simulink model "Bebop7_like6_but_spline_only_from_SP"  (R2018a)
settings: Solver=VariableStepAuto  StartTime=0.0  StopTime=20  FixedStep=.04  MaxStep=1.00  MinStep=0.005  RelTol=10  AbsTol=10
values from neighbouring files (symbols this model uses):
  flightplan = [dist,0,height,deg2rad(090) ... (first row only)    [compare_cubic_spline_1.m]    (also in initialize_race_realtime.m; initialize_race_realtime_backup_cubic.m; plot_sim.m = [ 4.348, -0.278, height, deg2rad(  0); test_b_spline.m)
  FOV = 1.05    [initialize_race_realtime.m]    (also in initialize_race_realtime_backup_cubic.m)
  g = 9.81    [initialize_race_no_realtime.m]    (also in initialize_race_realtime.m; initialize_race_realtime_backup_cubic.m; moving_average_rls_own.m = P(i-1)*meas*(lambda+meas*P(i-1)*meas)^-1)
  gate_size = 1.4    [initialize_race_realtime.m]    (also in initialize_race_realtime_backup_cubic.m)
  gates = sim_gates(:,:,1)    [eval_sim.m]    (also in initialize_race_realtime.m = [dist,0,height,deg2rad(110); initialize_race_realtime_backup_cubic.m = [dist,0,height,deg2rad(110); plot_sim.m)
  I = [1 0 0 ... (first row only)    [Bebop_sim_init.m]    (also in initialize_race_no_realtime.m; initialize_race_realtime.m; initialize_race_realtime_backup_cubic.m; moving_averge_rls_download.m = ones(1,N))
  init_std_dev = [1.0*ones(1,3),deg2rad(30)]    [initialize_race_realtime.m]    (also in initialize_race_realtime_backup_cubic.m)
  m = 0.68    [calc_plot_spline.m]    (also in calc_spline.m; compare_cubic_spline_1.m = vpasolve(e,r); compare_cubic_spline_2.m = r/3*(-sin(dp)+sqrt(sin(dp)^2-6*cos(dp)+6)); initialize_race_no_realtime.m = 2)
  max_rot_Z = (90)*pi/180    (= 1.57079632679)    [Bebop_sim_init.m]    (also in initialize_race_no_realtime.m = 1.0471975512; initialize_race_realtime.m; initialize_race_realtime_backup_cubic.m; run_batch1.m = list_agility(idx_agility)*max_rot_Z)
  max_theta_X = (40)*pi/180    (= 0.698131700798)    [Bebop_sim_init.m]    (also in initialize_race_no_realtime.m = 0.13962634016; initialize_race_realtime.m = 1.308996939; initialize_race_realtime_backup_cubic.m = 1.308996939; run_batch1.m = list_agility(idx_agility)*max_theta_X)
  max_theta_Y = (40)*pi/180    (= 0.698131700798)    [Bebop_sim_init.m]    (also in initialize_race_no_realtime.m = 0.13962634016; initialize_race_realtime.m = 1.308996939; initialize_race_realtime_backup_cubic.m = 1.308996939; run_batch1.m = list_agility(idx_agility)*max_theta_Y)
  max_v_Z = .5    (= 0.5)    [Bebop_sim_init.m]    (also in initialize_race_no_realtime.m = 1; initialize_race_realtime.m = 3; initialize_race_realtime_backup_cubic.m = 3; run_batch1.m = list_agility(idx_agility)*max_v_Z)
  max_vel = 1.5    [initialize_race_realtime.m]    (also in initialize_race_realtime_backup_cubic.m; run_batch1.m = list_speed(idx_speed); run_batch2.m = list_speed(idx_speed); run_batch3.m = list_speed(idx_speed))
  spline_init = [P0;P1;P2;P3]    [initialize_race_realtime.m]
  std_dev_factor = 1.0    (= 1)    [initialize_race_realtime.m]
  std_dev_switch = std_dev_factor/5    (= 0.2)    [initialize_race_realtime.m]
undefined symbols (not defined in the file or in its folder): fspecial, gray, Rec, SDTV
libraries: simulink x11, sharedtransform x11, visionanalysis x7, visiontextngfix x5, visiontransforms x3, aerolibactuator x2, aerolibutil x2, visionstatistics x2, visionconversions x2, shared6dof x1, vrlib x1, visionsinks x1
(part 1 of 3)
settings Model: EnablePacing=on  Creator=vinni  LastModifiedBy=lenny
settings SolverCC: MaxConsecutiveMinStep=99999  ShapePreserveControl=EnableAll  ZeroCrossAlgorithm=Adaptive
settings DebuggingCC: WriteAfterWriteMsg=EnableAllAsError  AlgebraicLoopMsg=error  IntegerOverflowMsg=error  ParameterUnderflowMsg=error  UniqueDataStoreMsg=error  NonBusSignalsTreatedAsBus=error  IntegerSaturationMsg=error
settings HardwareCC: ProdBitPerLong=64  ProdHWDeviceType=Intel->x86-64 (Linux 64)

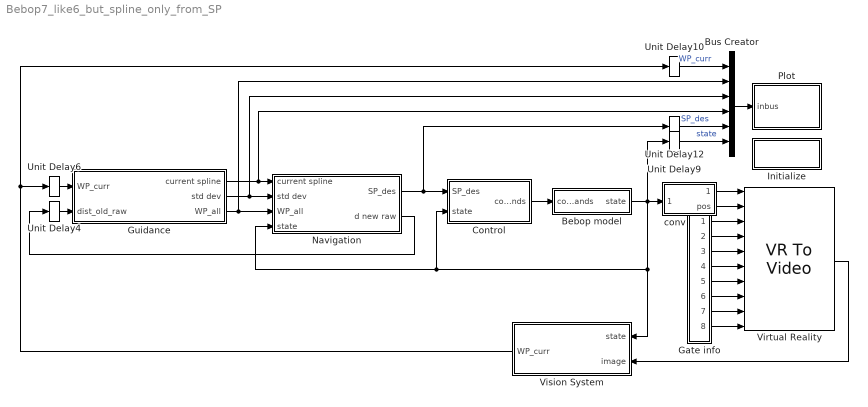
== system Bebop7_like6_but_spline_only_from_SP ==
  Bebop model : Subsystem
  Bus Creator : BusCreator  Inputs=6  OutDataTypeStr=Bus: PlotBus  NonVirtualBus=on
  Control : Subsystem
  Gate info : Subsystem
  Guidance : Subsystem
  Initialize : Subsystem  TreatAsAtomicUnit=on
  Navigation : Subsystem
  Plot : MATLAB Function  TreatAsAtomicUnit=on
  Unit Delay{4,6,9..10,12} (5 alike) : UnitDelay  SampleTime=-1
  Virtual Reality : vrlib/VR To Video  InstantiateOnLoad=on  SampleTime=0.075  ViewEnable=on  RemoteChange=off  RemoteView=off  FieldsWritten=drone.orientation.4.1.1.double#drone.position.3.1.1.double#G1.rotation.4.1.1.double#G1.translation.3.1.1.double#G2.rotation.4.1.1.double#G2.translation.3.1.1.double#G3.rotation.4.1.1.double#G3.translation.3.1.1.double#G4.rotation.4.1.1.double#G4.translation.3.1.1.double  WorldFileName=race_course.wrl  AutoView=off  VideoDimensions=1.5*[200 320]  AllowVariableSize=off  FigureProperties="{'Position', 'Name', 'Viewpoint', 'CameraBound', 'CameraDirection', 'CameraPosition', 'CameraUpVector', 'ZoomFactor', 'Antialiasing', 'Headlight', 'Lighting', 'NavPanel', 'Sound', 'StatusBar', 'Stereo3D', 'Stereo3DCameraOffset', 'Stereo3DHIT', 'ToolBar', 'Textures', 'Transparency', 'Triad', 'Wireframe', 'NavZones', 'NavMode', 'NavSpeed', 'CaptureFileFormat', 'CaptureFileName', 'Record2DCompressMethod', 'Record2DCompressQuality', 'Record2D', 'Record2DFileName', 'Record2DFPS'; [3.0000000000000000e+01   6.0000000000000000e+01   4.8000000000000000e+02   3.0000000000000000e+02], '', '_untitled_1', 'on', [0.0000000000000000e+00   0.0000000000000000e+00  -1.0000000000000000e+00], [0.0000000000000000e+00   0.0000000000000000e+00   0.0000000000000000e+00], [0.0000000000000000e+00   1.0000000000000000e+00   0.0000000000000000e+00], [1.0000000000000000e+00], 'on', 'on', 'on', 'none', 'on', 'off', 'off', [1.0000000149011612e-01], [0.0000000000000000e+00], 'off', 'on', 'on', 'none', 'off', 'off', 'fly', 'normal', 'tif', '%f_anim_%n.tif', 'auto', [7.5000000000000000e+01], 'off', '***video***', 'auto'}"
      settings: SourceProductName=Simulink 3D Animation  SourceProductBaseCode=VR
  Vision System : Subsystem
  conv : Subsystem
  wires:
  Vision System/1(WP_curr) -> Unit Delay10/1, Unit Delay6/1
  Virtual Reality/1 -> Vision System/2(image)
  Control/1(commands) -> Bebop model/1(commands)
  Unit Delay6/1 -> Guidance/1(WP_curr)
  Unit Delay4/1 -> Guidance/2(dist_old_raw)
  conv/1(axang) -> Virtual Reality/1
  Gate info/2(P1) -> Virtual Reality/4
  Gate info/4(P2) -> Virtual Reality/6
  Gate info/6(P3) -> Virtual Reality/8
  Gate info/8(P4) -> Virtual Reality/10
  Gate info/1(O1) -> Virtual Reality/3
  Gate info/3(O2) -> Virtual Reality/5
  Gate info/5(O3) -> Virtual Reality/7
  Gate info/7(O4) -> Virtual Reality/9
  Navigation/1(SP_des) -> Unit Delay12/1, Control/1(SP_des)
  Navigation/2(d new raw) -> Unit Delay4/1
  Bebop model/1(state) -> Vision System/1(state), Control/2(state), Navigation/4(state), Unit Delay9/1, conv/1(state)
  Bus Creator/1 -> Plot/1(inbus)
  Guidance/3(WP_all) -> Bus Creator/2, Navigation/3(WP_all)
  Guidance/2(std dev) -> Bus Creator/3, Navigation/2(std dev)
  Unit Delay9/1 -> Bus Creator/6  "state"
  Unit Delay10/1 -> Bus Creator/1  "WP_curr"
  Unit Delay12/1 -> Bus Creator/5  "SP_des"
  Guidance/1(current spline) -> Navigation/1(current spline), Bus Creator/4
  conv/2(pos) -> Virtual Reality/2

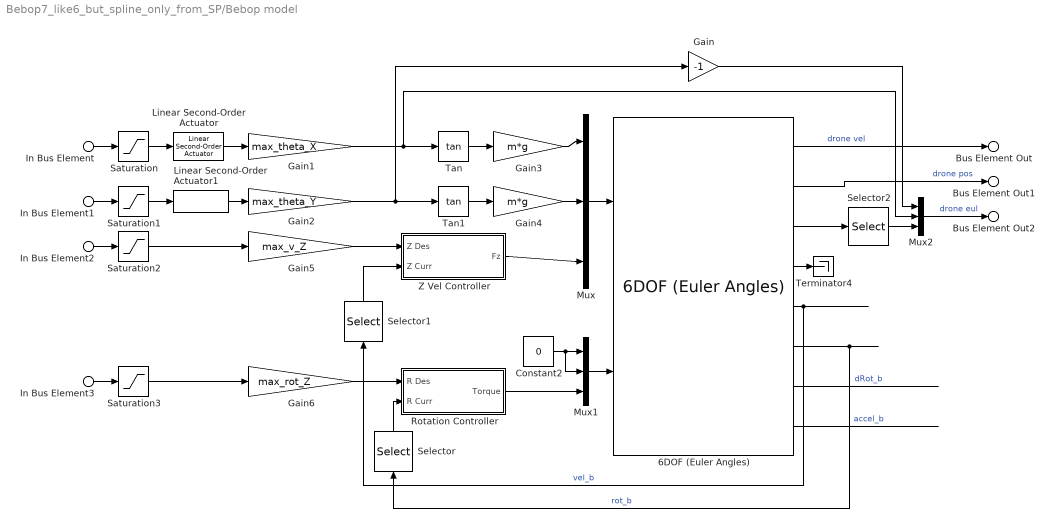
== system Bebop7_like6_but_spline_only_from_SP/Bebop model ==
  In Bus Element : Inport  PortName=commands  Element=pitch
  In Bus Element1 : Inport  PortName=commands  Element=roll
  In Bus Element2 : Inport  PortName=commands  Element=throttle
  In Bus Element3 : Inport  PortName=commands  Element=yaw
  6DOF (Euler Angles) : shared6dof/6DOF (Euler Angles)  units=Metric (MKS)  mtype=Fixed  rep=Euler Angles  xme_0=Initial_pos  Vm_0=Initial_vel_b  eul_0=Initial_ori  pm_0=[0 0 0]  mass_0=m  mass_e=0.5  mass_f=2.0  inertia=I  inertia_e=eye(3)  inertia_f=2*eye(3)  k_quat=1.0  vre_flag=on  abi_flag=off  aMode=0
      settings: SourceProductBaseCode=AE
  Constant2 : Constant  Value=0
  Gain : Gain  Gain=-1
  Gain1 : Gain  Gain=max_theta_X
  Gain2 : Gain  Gain=max_theta_Y
  Gain3 : Gain  Gain=m*g
  Gain4 : Gain  Gain=m*g
  Gain5 : Gain  Gain=max_v_Z
  Gain6 : Gain  Gain=max_rot_Z
  Linear Second-Order Actuator : aerolibactuator/Linear Second-Order Actuator  wn_fin=20  z_fin=1  fin_act_0=0  fin_act_vel=0
      settings: SourceProductName=Aerospace Blockset  SourceProductBaseCode=AE
  Linear Second-Order Actuator1 : aerolibactuator/Linear Second-Order Actuator  wn_fin=20  z_fin=1  fin_act_0=0  fin_act_vel=0
      settings: SourceProductName=Aerospace Blockset  SourceProductBaseCode=AE
  Mux : Mux  Inputs=3
  Mux1 : Mux  Inputs=3
  Mux2 : Mux  Inputs=3
  Rotation Controller : Subsystem
  Saturation{,1..3} (4 alike) : Saturate  UpperLimit=1  LowerLimit=-1
  Selector : Selector  InputPortWidth=3  IndexOptions=Index vector (dialog)  Indices=3  OutputSizes=1
  Selector1 : Selector  InputPortWidth=3  IndexOptions=Index vector (dialog)  Indices=3  OutputSizes=1
  Selector2 : Selector  InputPortWidth=3  IndexOptions=Index vector (dialog)  Indices=3  OutputSizes=1
  Tan : Trigonometry  Operator=tan
  Tan1 : Trigonometry  Operator=tan
  Terminator4 : Terminator
  Z Vel Controller : Subsystem
  Bus Element Out : Outport  PortName=state  Element=vel
  Bus Element Out1 : Outport  PortName=state  Element=pos
  Bus Element Out2 : Outport  PortName=state  Element=eul
  wires:
  6DOF (Euler Angles)/5 -> Selector1/1  "vel_b"
  Saturation/1 -> Linear Second-Order Actuator/1
  Tan1/1 -> Gain4/1
  In Bus Element3/1 -> Saturation3/1
  Linear Second-Order Actuator1/1 -> Gain2/1
  6DOF (Euler Angles)/8 -> ?  "accel_b"
  Z Vel Controller/1(Fz) -> Mux/3
  6DOF (Euler Angles)/1 -> Bus Element Out/1  "drone vel"
  Rotation Controller/1(Torque) -> Mux1/3
  Selector/1 -> Rotation Controller/2(R Curr)
  Selector1/1 -> Z Vel Controller/2(Z Curr)
  Gain3/1 -> Mux/1
  Saturation1/1 -> Linear Second-Order Actuator1/1
  6DOF (Euler Angles)/3 -> Selector2/1
  In Bus Element2/1 -> Saturation2/1
  Gain1/1 -> Mux2/2, Tan/1
  Mux/1 -> 6DOF (Euler Angles)/1
  Gain5/1 -> Z Vel Controller/1(Z Des)
  In Bus Element1/1 -> Saturation1/1
  Tan/1 -> Gain3/1
  Gain/1 -> Mux2/1
  6DOF (Euler Angles)/4 -> Terminator4/1
  Constant2/1 -> Mux1/2, Mux1/1
  Saturation2/1 -> Gain5/1
  Gain2/1 -> Tan1/1, Gain/1
  Saturation3/1 -> Gain6/1
  Linear Second-Order Actuator/1 -> Gain1/1
  Mux1/1 -> 6DOF (Euler Angles)/2
  Gain6/1 -> Rotation Controller/1(R Des)
  Gain4/1 -> Mux/2
  In Bus Element/1 -> Saturation/1
  6DOF (Euler Angles)/6 -> Selector/1  "rot_b"
  6DOF (Euler Angles)/7 -> ?  "dRot_b"
  Selector2/1 -> Mux2/3
  6DOF (Euler Angles)/2 -> Bus Element Out1/1  "drone pos"
  Mux2/1 -> Bus Element Out2/1  "drone eul"

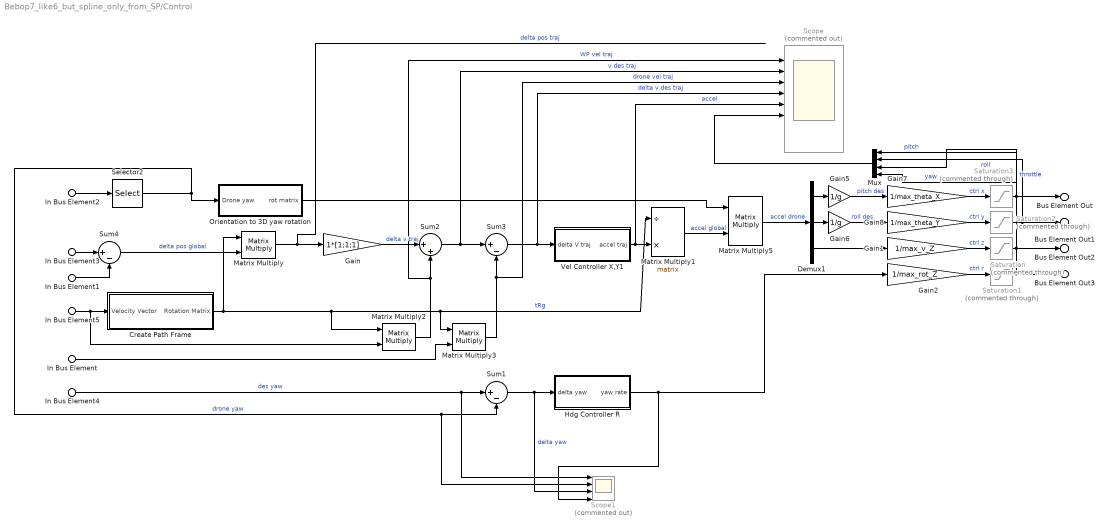
== system Bebop7_like6_but_spline_only_from_SP/Control ==
  In Bus Element5 : Inport  PortName=SP_des  Element=vel
  In Bus Element3 : Inport  PortName=SP_des  Element=pos
  In Bus Element4 : Inport  PortName=SP_des  Element=yaw
  In Bus Element : Inport  Port=2  PortName=state  Element=vel
  In Bus Element1 : Inport  Port=2  PortName=state  Element=pos
  In Bus Element2 : Inport  Port=2  PortName=state  Element=eul
  Create Path Frame : Subsystem
  Demux1 : Demux  Outputs=3
  Gain : Gain  Gain=1*[1;1;1]
  Gain1 : Gain  Gain=1/max_v_Z
  Gain2 : Gain  Gain=1/max_rot_Z
  Gain5 : Gain  Gain=1/g
  Gain6 : Gain  Gain=1/g
  Gain7 : Gain  Gain=1/max_theta_X
  Gain8 : Gain  Gain=1/max_theta_Y
  Hdg Controller R : Subsystem
  Matrix Multiply{,2..3,5} (4 alike) : Product  Inputs=**  Multiplication=Matrix(*)
  Matrix Multiply1 : Product  Inputs=/*  Multiplication=Matrix(*)
  Mux : Mux
  Orientation to 3D yaw rotation : Subsystem
  Saturation{,1..3} (4 alike) : Saturate  Commented=through  UpperLimit=1  LowerLimit=-1
  Scope : Scope  Commented=on  NumInputPorts=10
  Scope1 : Scope  Commented=on  NumInputPorts=4
  Selector2 : Selector  IndexMode=Zero-based  InputPortWidth=3  IndexOptions=Index vector (dialog)  Indices=2  OutputSizes=1
  Sum1 : Sum  Inputs=|+-
  Sum2 : Sum  Inputs=|++
  Sum3 : Sum  Inputs=|+-
  Sum4 : Sum  Inputs=|+-
  Vel Controller X,Y1 : Subsystem
  Bus Element Out : Outport  PortName=commands  Element=pitch
  Bus Element Out1 : Outport  PortName=commands  Element=roll
  Bus Element Out2 : Outport  PortName=commands  Element=throttle
  Bus Element Out3 : Outport  PortName=commands  Element=yaw
  wires:
  Saturation1/1 -> Bus Element Out3/1, Mux/4  "yaw"
  Saturation3/1 -> Bus Element Out/1, Mux/1  "pitch"
  Saturation2/1 -> Bus Element Out1/1, Mux/2  "roll"
  Saturation/1 -> Bus Element Out2/1, Mux/3  "throttle"
  In Bus Element4/1 -> Scope1/1, Sum1/1  "des yaw"
  In Bus Element3/1 -> Sum4/1
  In Bus Element5/1 -> Matrix Multiply2/2, Create Path Frame/1(Velocity Vector)
  Selector2/1 -> Scope1/2, Sum1/2, Orientation to 3D yaw rotation/1(Drone yaw)  "drone yaw"
  Gain7/1 -> Saturation3/1  "ctrl x"
  Demux1/3 -> Gain1/1
  Hdg Controller R/1(yaw rate) -> Scope1/4, Gain2/1
  Demux1/2 -> Gain6/1
  Mux/1 -> Scope/7
  Gain6/1 -> Gain8/1  "roll des"
  Sum3/1 -> Scope/5, Vel Controller X,Y1/1(delta V traj)  "delta v des traj"
  Matrix Multiply2/1 -> Scope/2, Sum2/2  "WP vel traj"
  Sum4/1 -> Matrix Multiply/2  "delta pos global"
  Matrix Multiply3/1 -> Scope/4, Sum3/2  "drone vel traj"
  Demux1/1 -> Gain5/1
  Gain1/1 -> Saturation/1  "ctrl z"
  Matrix Multiply/1 -> Gain/1  "delta pos traj"
  Gain5/1 -> Gain7/1  "pitch des"
  Vel Controller X,Y1/1(accel traj) -> Scope/6, Matrix Multiply1/2  "accel"
  Matrix Multiply5/1 -> Demux1/1  "accel drone"
  Orientation to 3D yaw rotation/1(rot matrix) -> Matrix Multiply5/1
  Gain8/1 -> Saturation2/1  "ctrl y"
  In Bus Element1/1 -> Sum4/2
  Create Path Frame/1(Rotation Matrix) -> Matrix Multiply/1, Matrix Multiply2/1, Matrix Multiply1/1, Matrix Multiply3/1  "tRg"
  Gain2/1 -> Saturation1/1  "ctrl r"
  In Bus Element/1 -> Matrix Multiply3/2
  Gain/1 -> Sum2/1  "delta v traj"
  Sum2/1 -> Scope/3, Sum3/1  "v des traj"
  Matrix Multiply1/1 -> Matrix Multiply5/2  "accel global"
  Sum1/1 -> Scope1/3, Hdg Controller R/1(delta yaw)  "delta yaw"
  In Bus Element2/1 -> Selector2/1

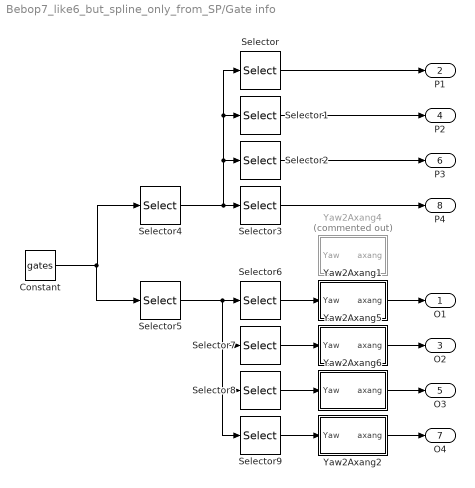
== system Bebop7_like6_but_spline_only_from_SP/Gate info ==
  Constant : Constant  Value=gates
  Selector : Selector  NumberOfDimensions=2  IndexMode=Zero-based  InputPortWidth=3  IndexOptions=Index vector (dialog),Select all  Indices=0,1  OutputSizes=1,1
  Selector1 : Selector  NumberOfDimensions=2  IndexMode=Zero-based  InputPortWidth=3  IndexOptions=Index vector (dialog),Select all  Indices=1,1  OutputSizes=1,1
  Selector2 : Selector  NumberOfDimensions=2  IndexMode=Zero-based  InputPortWidth=3  IndexOptions=Index vector (dialog),Select all  Indices=2,1  OutputSizes=1,1
  Selector3 : Selector  NumberOfDimensions=2  IndexMode=Zero-based  InputPortWidth=3  IndexOptions=Index vector (dialog),Select all  Indices=3,1  OutputSizes=1,1
  Selector4 : Selector  NumberOfDimensions=2  IndexMode=Zero-based  InputPortWidth=3  IndexOptions=Select all,Index vector (dialog)  Indices=4,[0 1 2]  OutputSizes=1,1
  Selector5 : Selector  NumberOfDimensions=2  IndexMode=Zero-based  InputPortWidth=3  IndexOptions=Select all,Index vector (dialog)  Indices=4,3  OutputSizes=1,1
  Selector6 : Selector  NumberOfDimensions=2  IndexMode=Zero-based  InputPortWidth=3  IndexOptions=Index vector (dialog),Select all  Indices=0,1  OutputSizes=1,1
  Selector7 : Selector  NumberOfDimensions=2  IndexMode=Zero-based  InputPortWidth=3  IndexOptions=Index vector (dialog),Select all  Indices=1,1  OutputSizes=1,1
  Selector8 : Selector  NumberOfDimensions=2  IndexMode=Zero-based  InputPortWidth=3  IndexOptions=Index vector (dialog),Select all  Indices=2,1  OutputSizes=1,1
  Selector9 : Selector  NumberOfDimensions=2  IndexMode=Zero-based  InputPortWidth=3  IndexOptions=Index vector (dialog),Select all  Indices=3,1  OutputSizes=1,1
  Yaw2Axang1 : Subsystem
  Yaw2Axang2 : Subsystem
  Yaw2Axang4 : Subsystem  Commented=on
  Yaw2Axang5 : Subsystem
  Yaw2Axang6 : Subsystem
  O1 : Outport
  P1 : Outport  Port=2
  O2 : Outport  Port=3
  P2 : Outport  Port=4
  O3 : Outport  Port=5
  P3 : Outport  Port=6
  O4 : Outport  Port=7
  P4 : Outport  Port=8
  wires:
  Selector/1 -> P1/1
  Selector3/1 -> P4/1
  Selector2/1 -> P3/1
  Selector4/1 -> Selector1/1, Selector/1, Selector2/1, Selector3/1
  Selector1/1 -> P2/1
  Constant/1 -> Selector5/1, Selector4/1
  Selector5/1 -> Selector9/1, Selector8/1, Selector7/1, Selector6/1
  Selector6/1 -> Yaw2Axang1/1(Yaw)
  Selector7/1 -> Yaw2Axang5/1(Yaw)
  Selector8/1 -> Yaw2Axang6/1(Yaw)
  Selector9/1 -> Yaw2Axang2/1(Yaw)
  Yaw2Axang1/1(axang) -> O1/1
  Yaw2Axang5/1(axang) -> O2/1
  Yaw2Axang6/1(axang) -> O3/1
  Yaw2Axang2/1(axang) -> O4/1

== system Bebop7_like6_but_spline_only_from_SP/Guidance ==
  Bus Element In1 : Inport  PortName=WP_curr  Element=eul
  Bus Element In : Inport  PortName=WP_curr  Element=pos
  dist_old_raw : Inport  Port=2
  Constant : Constant  Value=init_std_dev
  Scope : Scope  Commented=on
  Unit Delay1 : UnitDelay  InitialCondition=init_std_dev  SampleTime=-1
  Unit Delay2 : UnitDelay  SampleTime=-1
  Unit Delay3 : UnitDelay  InitialCondition=flightplan  SampleTime=-1
  Unit Delay4 : UnitDelay  InitialCondition=spline_init  SampleTime=-1
  create_spline : MATLAB Function  TreatAsAtomicUnit=on
  filter_WP_moving_av : MATLAB Function  TreatAsAtomicUnit=on
  select_WP : MATLAB Function  TreatAsAtomicUnit=on
  current spline : Outport
  std dev : Outport  Port=2
  Out Bus Element : Outport  Port=3  PortName=WP_all  Element=list
  Out Bus Element1 : Outport  Port=3  PortName=WP_all  Element=idx
  wires:
  Bus Element In1/1 -> filter_WP_moving_av/6(WP_current_eul)
  create_spline/1(current_spline) -> Scope/1, Unit Delay4/1, current spline/1  "current spline"
  Bus Element In/1 -> filter_WP_moving_av/5(WP_current_pos)
  select_WP/1(WP_average) -> create_spline/2(WP_average)
  Unit Delay3/1 -> filter_WP_moving_av/1(WP_list_in)
  Unit Delay2/1 -> filter_WP_moving_av/2(WP_idx_in)
  Unit Delay1/1 -> filter_WP_moving_av/3(WP_std_dev_in)
  Constant/1 -> filter_WP_moving_av/7(init_std_dev)
  filter_WP_moving_av/3(WP_std_dev_out) -> Unit Delay1/1, std dev/1, create_spline/3(std_dev)  "std dev"
  filter_WP_moving_av/2(WP_idx_out) -> Out Bus Element1/1, select_WP/2(WP_idx), Unit Delay2/1
  filter_WP_moving_av/1(WP_list_out) -> select_WP/1(WP_list), Out Bus Element/1, Unit Delay3/1
  dist_old_raw/1 -> create_spline/4(d_old_raw), filter_WP_moving_av/4(dist_old_raw)  "d_old_raw"
  Unit Delay4/1 -> create_spline/1(old_spline)

== system Bebop7_like6_but_spline_only_from_SP/Initialize ==
  Event Listener : EventListener  DisableCoverage=on  EventName=reset
  reset_plot : MATLAB Function  TreatAsAtomicUnit=on

== system Bebop7_like6_but_spline_only_from_SP/Navigation ==
  current spline : Inport
  std dev : Inport  Port=2
  In Bus Element : Inport  Port=3  PortName=WP_all  Element=list
  In Bus Element3 : Inport  Port=3  PortName=WP_all  Element=idx
  In Bus Element1 : Inport  Port=4  PortName=state  Element=pos
  Scope : Scope  Commented=on  NumInputPorts=5
  calc v : Subsystem
  calculate desired : Subsystem
  get WPts : Subsystem
  select d : MATLAB Function  TreatAsAtomicUnit=on
  set position : Subsystem
  Bus Element Out : Outport  PortName=SP_des  Element=pos
  Bus Element Out1 : Outport  PortName=SP_des  Element=vel
  Bus Element Out2 : Outport  PortName=SP_des  Element=yaw
  d new raw : Outport  Port=2
  wires:
  calculate desired/2(WP vel des) -> Bus Element Out1/1
  current spline/1 -> calc v/1(current spline), calculate desired/2(current spline), set position/1(current spline)
  calculate desired/1(yaw) -> Bus Element Out2/1
  In Bus Element1/1 -> calculate desired/5(drone current pos), calc v/3(drone current pos)
  set position/2(d new raw) -> d new raw/1
  get WPts/3(WP next) -> calculate desired/7(WP next)
  get WPts/2(WP this) -> calc v/4(WP this), calculate desired/6(WP this)
  std dev/1 -> select d/2(std_dev), calculate desired/1(std dev), calc v/2(std dev)
  set position/1(d old1) -> select d/1("d_old "), Scope/4, calculate desired/3(d)
  calculate desired/3(pos) -> calc v/5(drone desired pos), Bus Element Out/1
  calc v/1(velocity) -> Scope/2, calculate desired/4(vel), set position/2(velocity)
  In Bus Element/1 -> get WPts/1(list)
  In Bus Element3/1 -> get WPts/2(idx)
  select d/1(d_old) -> set position/3(d old), calc v/6(d)

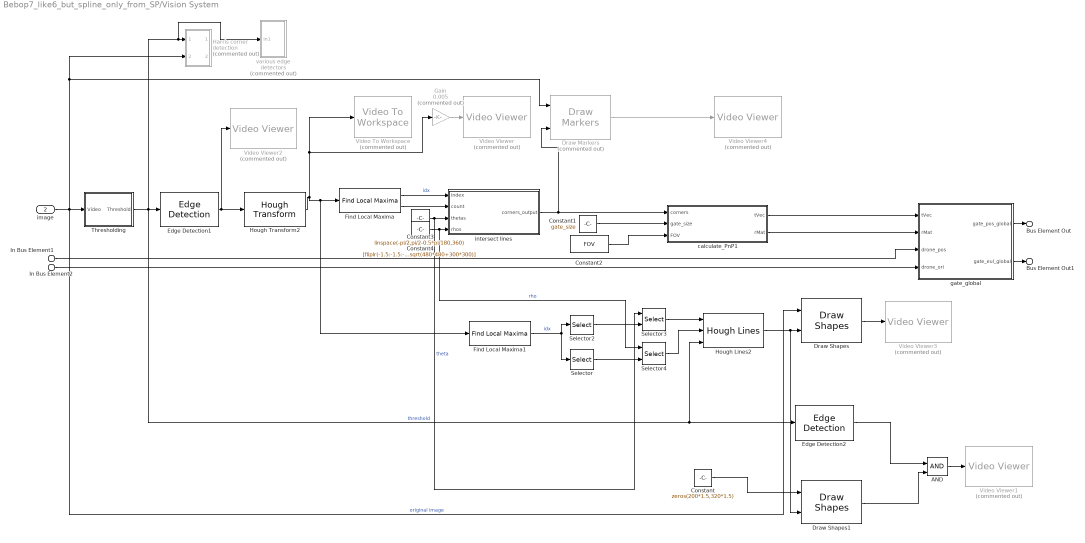
== system Bebop7_like6_but_spline_only_from_SP/Vision System ==
  In Bus Element1 : Inport  PortName=state  Element=pos
  In Bus Element2 : Inport  PortName=state  Element=eul
  image : Inport  Port=2
  AND : Logic  IconShape=distinctive  AllPortsSameDT=off  OutDataTypeStr=boolean
  Constant : Constant  Value=zeros(200*1.5,320*1.5)
  Constant1 : Constant  Value=gate_size
  Constant2 : Constant  Value=FOV
  Constant3 : Constant  Value=linspace(-pi/2,pi/2-0.5*pi/180,360)
  Constant4 : Constant  Value=[fliplr(-1.5:-1.5:-sqrt(480*480+300*300)), 0:1.5:sqrt(480*480+300*300)]
  Draw Markers : visiontextngfix/Draw Markers  Commented=on  shape=X-mark  size=10  fill=on  fillClrSource=Specify via dialog  display=User-specified value  intensity=200  color=[255 0 0]  opacity=0.6  viewport=Entire image  antialiasing=off  inType=Obsolete  imagePorts=One multidimensional signal  prodOutputMode=Binary point scaling  prodOutputWordLength=32  prodOutputFracLength=14  memoryMode=Specify word length  memoryWordLength=16  memoryFracLength=14  roundingMode=Floor  overflowMode=off
      settings: SourceProductName=Computer Vision System Toolbox  SourceProductBaseCode=VP
  Draw Shapes : visiontextngfix/Draw Shapes  shape=Lines  fill=off  lineWidth=1  fillClrSource=Specify via dialog  display=White  intensity=200  color=[200 255 100]  opacity=0.6  viewport=Entire image  antialiasing=off  inType=Obsolete  imagePorts=One multidimensional signal  prodOutputMode=Binary point scaling  prodOutputWordLength=32  prodOutputFracLength=14  memoryMode=Specify word length  memoryWordLength=16  memoryFracLength=15  roundingMode=Floor  overflowMode=off
      settings: SourceProductName=Computer Vision System Toolbox
  Draw Shapes1 : visiontextngfix/Draw Shapes  shape=Lines  fill=off  lineWidth=4  fillClrSource=Specify via dialog  display=White  intensity=200  color=[200 255 100]  opacity=0.6  viewport=Entire image  antialiasing=off  inType=Obsolete  imagePorts=One multidimensional signal  prodOutputMode=Binary point scaling  prodOutputWordLength=32  prodOutputFracLength=14  memoryMode=Specify word length  memoryWordLength=16  memoryFracLength=14  roundingMode=Floor  overflowMode=off
      settings: SourceProductName=Computer Vision System Toolbox
  Edge Detection1 : visionanalysis/Edge Detection  method=Sobel  outputType=Binary image  userDefinedThreshold=off  thresholdSource=Input port  threshold=20  thresholdTuning=20  edgeThinning=on  threshold_canny=[0.25 0.60]  autoPercent=70  sigma=1  roundingMode=Floor  overflowMode=off  prodOutputMode=Binary point scaling  prodOutputWordLength=32  prodOutputFracLength=8  prodOutputSlope=2^-8  accumSlope=2^-8  outputSlope=2^-4
      settings: SourceProductName=Computer Vision System Toolbox  SourceProductBaseCode=VP
  Edge Detection2 : visionanalysis/Edge Detection  method=Sobel  outputType=Binary image  userDefinedThreshold=off  thresholdSource=Input port  threshold=20  thresholdTuning=20  edgeThinning=off  threshold_canny=[0.25 0.60]  autoPercent=70  sigma=1  roundingMode=Floor  overflowMode=off  prodOutputMode=Binary point scaling  prodOutputWordLength=32  prodOutputFracLength=8  prodOutputSlope=2^-8  accumSlope=2^-8  outputSlope=2^-4
      settings: SourceProductName=Computer Vision System Toolbox  SourceProductBaseCode=VP
  Find Local Maxima : visionstatistics/Find Local Maxima  num_peaks=8  nhood_size=[7 15]  src_thresh=Obsolete9b  src_thresh_inuse=Specify via dialog  threshold=100  inputIsHough=on  dt_peak=uint32  isOutVarDim=off  dt_count=uint32
      settings: SourceProductName=Computer Vision System Toolbox  SourceProductBaseCode=VP
  Find Local Maxima1 : visionstatistics/Find Local Maxima  num_peaks=16  nhood_size=[7 15]  src_thresh=Obsolete9b  src_thresh_inuse=Specify via dialog  threshold=100  inputIsHough=on  dt_peak=uint32  isOutVarDim=on  dt_count=uint32
      settings: SourceProductName=Computer Vision System Toolbox  SourceProductBaseCode=VP
  Gain : Gain  Commented=on  Gain=0.005
  Harris corner detection : Subsystem  Commented=on
  Hough Lines2 : visiontransforms/Hough Lines  sineCompMethod=Trigonometric function  thetaRes=pi/180  firstCoeffMode=Specify word length  firstCoeffWordLength=16  firstCoeffFracLength=15  prodOutputMode=Binary point scaling  prodOutputWordLength=32  prodOutputFracLength=16  roundingMode=Nearest  overflowMode=on
      settings: SourceProductName=Computer Vision System Toolbox  SourceProductBaseCode=VP
  Hough Transform2 : visiontransforms/Hough Transform  theta_res=0.5*pi/180  rho_res=1.5  out_theta_rho=off  outdtmode=double  firstCoeffMode=Binary point scaling  firstCoeffWordLength=16  firstCoeffFracLength=14  secondCoeffMode=Binary point scaling  secondCoeffWordLength=32  secondCoeffFracLength=16  outputMode=Binary point scaling  outputWordLength=16  outputFracLength=0  accumMode=Binary point scaling  accumWordLength=32  accumFracLength=20  prodOutputMode=Binary point scaling  prodOutputWordLength=32  prodOutputFracLength=20  memoryMode=Binary point scaling  memoryWordLength=32  memoryFracLength=16  roundingMode=Nearest  overflowMode=on
      settings: SourceProductName=Computer Vision System Toolbox  SourceProductBaseCode=VP
  Selector : Selector  NumberOfDimensions=2  IndexMode=Zero-based  InputPortWidth=2  IndexOptions=Select all,Index vector (dialog)  Indices=2,1  OutputSizes=1,1
  Selector2 : Selector  NumberOfDimensions=2  IndexMode=Zero-based  InputPortWidth=2  IndexOptions=Select all,Index vector (dialog)  Indices=1,0  OutputSizes=1,1
  Selector3 : Selector  NumberOfDimensions=2  InputPortWidth=3  IndexOptions=Select all,Index vector (port)  Indices=[1 3],1  OutputSizes=1,1
  Selector4 : Selector  NumberOfDimensions=2  InputPortWidth=3  IndexOptions=Select all,Index vector (port)  Indices=[1 3],1  OutputSizes=1,1
  Thresholding : Subsystem
  Video To Workspace : visionsinks/Video To Workspace  Commented=on  VariableName=vout  NumInputs=1  DataLimit=10  DecimationFactor=1  LogFi=off  InPortLabels=R|G|B
      settings: SourceProductName=Computer Vision System Toolbox  SourceProductBaseCode=VP
  Video Viewer : VideoViewer  Commented=on  colormapValue=gray(256)  FigPos=[66 898 768 765]
  Video Viewer1 : VideoViewer  Commented=on  colormapValue=gray(256)  FigPos=[983 1078 938 945]
  Video Viewer2 : VideoViewer  Commented=on  colormapValue=gray(256)  FigPos=[993 1078 928 945]
  Video Viewer3 : VideoViewer  Commented=on  colormapValue=gray(256)  FigPos=[993 1078 928 945]
  Video Viewer4 : VideoViewer  Commented=on  colormapValue=gray(256)  FigPos=[983 1078 938 945]
  calculate_PnP1 : MATLAB Function  TreatAsAtomicUnit=on
  gate_global : MATLAB Function  TreatAsAtomicUnit=on
  intersect lines : MATLAB Function  TreatAsAtomicUnit=on
  various edge detectors : Subsystem  Commented=on
  Bus Element Out : Outport  PortName=WP_curr  Element=pos
  Bus Element Out1 : Outport  PortName=WP_curr  Element=eul
  wires:
  Selector/1 -> Selector4/2
  Find Local Maxima/1 -> intersect lines/1(index)  "idx"
  Selector3/1 -> Hough Lines2/1
  Selector4/1 -> Hough Lines2/2
  Draw Shapes/1 -> Video Viewer3/1
  Hough Lines2/1 -> Draw Shapes1/2, Draw Shapes/2
  Selector2/1 -> Selector3/2
  Edge Detection1/1 -> Video Viewer2/1, Hough Transform2/1
  Gain/1 -> Video Viewer/1
  Draw Markers/1 -> Video Viewer4/1
  Constant3/1 -> intersect lines/3(thetas), Selector3/1  "theta"
  Constant4/1 -> Selector4/1, intersect lines/4(rhos)  "rho"
  image/1 -> Draw Shapes/1, Harris corner detection/2(original), Draw Markers/1, Thresholding/1("Video ")  "original image"
  Thresholding/1(Threshold) -> Hough Lines2/3, Edge Detection2/1, Harris corner detection/1(hreshold), various edge detectors/1(In1), Edge Detection1/1  "threshold"
  Constant1/1 -> calculate_PnP1/2(gate_size)
  calculate_PnP1/1(tVec) -> gate_global/1(tVec)
  calculate_PnP1/2(rMat) -> gate_global/2(rMat)
  Constant2/1 -> calculate_PnP1/3(FOV)
  In Bus Element2/1 -> gate_global/4(drone_ori)
  In Bus Element1/1 -> gate_global/3(drone_pos)
  gate_global/2(gate_eul_global) -> Bus Element Out1/1
  gate_global/1(gate_pos_global) -> Bus Element Out/1
  Hough Transform2/1 -> Find Local Maxima1/1, Find Local Maxima/1, Gain/1, Video To Workspace/1
  Find Local Maxima/2 -> intersect lines/2(count)
  intersect lines/1(corners_output) -> Draw Markers/2, calculate_PnP1/1(corners)
  Find Local Maxima1/1 -> Selector2/1, Selector/1  "idx"
  Draw Shapes1/1 -> AND/2
  Constant/1 -> Draw Shapes1/1
  AND/1 -> Video Viewer1/1
  Edge Detection2/1 -> AND/1

== system Bebop7_like6_but_spline_only_from_SP/conv ==
  In Bus Element : Inport  PortName=state  Element=eul
  In Bus Element1 : Inport  PortName=state  Element=pos
  global2strange drone : Subsystem
  axang : Outport
  pos : Outport  Port=2
  wires:
  In Bus Element/1 -> global2strange drone/1(euler global)
  global2strange drone/1(axang strange) -> axang/1
  In Bus Element1/1 -> pos/1

== system Bebop7_like6_but_spline_only_from_SP/Bebop model/Rotation Controller ==
  R Des : Inport
  R Curr : Inport  Port=2
  Gain : Gain  Gain=I(3,3)
  PID Controller : simulink/Continuous/PID Controller  Controller=PID  TimeDomain=Continuous-time  SampleTime=-1  IntegratorMethod=Forward Euler  FilterMethod=Forward Euler  Form=Parallel  UseFilter=on  ControllerParametersSource=internal  P=10  I=.3  D=.1  N=100  InitialConditionSource=internal  InitialConditionForIntegrator=0  InitialConditionForFilter=0  ExternalReset=none  LimitOutput=off  UpperSaturationLimit=inf  LowerSaturationLimit=-inf  LinearizeAsGain=on  AntiWindupMode=none  Kb=1  TrackingMode=off  Kt=1  PParamMin=[]  PParamMax=[]  IParamMin=[]  IParamMax=[]  DParamMin=[]  DParamMax=[]  NParamMin=[]  NParamMax=[]  KbParamMin=[]  KbParamMax=[]  KtParamMin=[]  KtParamMax=[]  POutMin=[]  POutMax=[]  IOutMin=[]  IOutMax=[]  DOutMin=[]  DOutMax=[]  NOutMin=[]  NOutMax=[]  KbOutMin=[]  KbOutMax=[]  KtOutMin=[]  KtOutMax=[]  IntegratorOutMin=[]  IntegratorOutMax=[]  FilterOutMin=[]  FilterOutMax=[]  SumOutMin=[]  SumOutMax=[]  SumI1OutMin=[]  SumI1OutMax=[]  SumI2OutMin=[]  SumI2OutMax=[]  SumI3OutMin=[]  SumI3OutMax=[]  SumDOutMin=[]  SumDOutMax=[]  SaturationOutMin=[]  SaturationOutMax=[]  IntegratorContinuousStateAttributes=''  IntegratorStateMustResolveToSignalObject=off  IntegratorRTWStateStorageClass=Auto  FilterContinuousStateAttributes=''  FilterStateMustResolveToSignalObject=off  FilterRTWStateStorageClass=Auto  DifferentiatorICPrevScaledInput=0  DifferentiatorOutMin=[]  DifferentiatorOutMax=[]  FilterDiffOutCoefMin=[]  FilterDiffOutCoefMax=[]  SumDenOutMin=[]  SumDenOutMax=[]  SumNumOutMin=[]  SumNumOutMax=[]  ReciprocalOutMin=[]  ReciprocalOutMax=[]  DivideOutMin=[]  DivideOutMax=[]  TunerSelectOption=Transfer Function Based (PID Tuner App)
  Scope : Scope  NumInputPorts=2
  Sum : Sum  Inputs=|+-
  Torque : Outport
  wires:
  R Des/1 -> Scope/1, Sum/1  "R Des"
  Sum/1 -> PID Controller/1
  R Curr/1 -> Scope/2, Sum/2  "R Curr"
  Gain/1 -> Torque/1
  PID Controller/1 -> Gain/1

== system Bebop7_like6_but_spline_only_from_SP/Bebop model/Z Vel Controller ==
  Z Des : Inport
  Z Curr : Inport  Port=2
  Gain : Gain  Gain=m
  PID Controller : simulink/Continuous/PID Controller  Controller=PID  TimeDomain=Continuous-time  SampleTime=-1  IntegratorMethod=Forward Euler  FilterMethod=Forward Euler  Form=Parallel  UseFilter=on  ControllerParametersSource=internal  P=5  I=.15  D=.1  N=100  InitialConditionSource=internal  InitialConditionForIntegrator=0  InitialConditionForFilter=0  ExternalReset=none  LimitOutput=off  UpperSaturationLimit=inf  LowerSaturationLimit=-inf  LinearizeAsGain=on  AntiWindupMode=none  Kb=1  TrackingMode=off  Kt=1  PParamMin=[]  PParamMax=[]  IParamMin=[]  IParamMax=[]  DParamMin=[]  DParamMax=[]  NParamMin=[]  NParamMax=[]  KbParamMin=[]  KbParamMax=[]  KtParamMin=[]  KtParamMax=[]  POutMin=[]  POutMax=[]  IOutMin=[]  IOutMax=[]  DOutMin=[]  DOutMax=[]  NOutMin=[]  NOutMax=[]  KbOutMin=[]  KbOutMax=[]  KtOutMin=[]  KtOutMax=[]  IntegratorOutMin=[]  IntegratorOutMax=[]  FilterOutMin=[]  FilterOutMax=[]  SumOutMin=[]  SumOutMax=[]  SumI1OutMin=[]  SumI1OutMax=[]  SumI2OutMin=[]  SumI2OutMax=[]  SumI3OutMin=[]  SumI3OutMax=[]  SumDOutMin=[]  SumDOutMax=[]  SaturationOutMin=[]  SaturationOutMax=[]  IntegratorContinuousStateAttributes=''  IntegratorStateMustResolveToSignalObject=off  IntegratorRTWStateStorageClass=Auto  FilterContinuousStateAttributes=''  FilterStateMustResolveToSignalObject=off  FilterRTWStateStorageClass=Auto  DifferentiatorICPrevScaledInput=0  DifferentiatorOutMin=[]  DifferentiatorOutMax=[]  FilterDiffOutCoefMin=[]  FilterDiffOutCoefMax=[]  SumDenOutMin=[]  SumDenOutMax=[]  SumNumOutMin=[]  SumNumOutMax=[]  ReciprocalOutMin=[]  ReciprocalOutMax=[]  DivideOutMin=[]  DivideOutMax=[]  TunerSelectOption=Transfer Function Based (PID Tuner App)
  Scope : Scope  NumInputPorts=2
  Sum : Sum  Inputs=|+-
  Fz : Outport
  wires:
  Z Des/1 -> Scope/1, Sum/1  "Z Des"
  Z Curr/1 -> Scope/2, Sum/2  "Z Curr"
  Sum/1 -> PID Controller/1
  Gain/1 -> Fz/1
  PID Controller/1 -> Gain/1

== system Bebop7_like6_but_spline_only_from_SP/Control/Create Path Frame ==
  Velocity Vector : Inport
  Invert 3x3 Matrix : aerolibutil/Invert  3x3 Matrix
  Make X Vector : Subsystem
  Make Y Vector : Subsystem
  Make Z Vector : Subsystem
  Matrix Concatenate : Concatenate  NumInputs=3  Mode=Multidimensional array  ConcatenateDimension=2
  Rotation Matrix : Outport
  wires:
  Velocity Vector/1 -> Make Z Vector/1(Velocity Vector), Make X Vector/1(Velocity Vector), Make Y Vector/1(Velocity Vector)
  Make Y Vector/1(Y Vector) -> Matrix Concatenate/2
  Make X Vector/1(X Vector) -> Matrix Concatenate/1
  Make Z Vector/1(Z Vector) -> Matrix Concatenate/3
  Matrix Concatenate/1 -> Invert 3x3 Matrix/1
  Invert 3x3 Matrix/1 -> Rotation Matrix/1

== system Bebop7_like6_but_spline_only_from_SP/Control/Hdg Controller R ==
  delta yaw : Inport
  Atan2 : Trigonometry  Operator=atan2
  Cos : Trigonometry  Operator=sincos
  PID Controller 0.075 : simulink/Continuous/PID Controller  Controller=PID  TimeDomain=Continuous-time  SampleTime=-1  IntegratorMethod=Forward Euler  FilterMethod=Forward Euler  Form=Parallel  UseFilter=on  ControllerParametersSource=internal  P=9  I=0  D=.9  N=100  InitialConditionSource=internal  InitialConditionForIntegrator=0  InitialConditionForFilter=0  ExternalReset=none  LimitOutput=off  UpperSaturationLimit=inf  LowerSaturationLimit=-inf  LinearizeAsGain=on  AntiWindupMode=none  Kb=1  TrackingMode=off  Kt=1  PParamMin=[]  PParamMax=[]  IParamMin=[]  IParamMax=[]  DParamMin=[]  DParamMax=[]  NParamMin=[]  NParamMax=[]  KbParamMin=[]  KbParamMax=[]  KtParamMin=[]  KtParamMax=[]  POutMin=[]  POutMax=[]  IOutMin=[]  IOutMax=[]  DOutMin=[]  DOutMax=[]  NOutMin=[]  NOutMax=[]  KbOutMin=[]  KbOutMax=[]  KtOutMin=[]  KtOutMax=[]  IntegratorOutMin=[]  IntegratorOutMax=[]  FilterOutMin=[]  FilterOutMax=[]  SumOutMin=[]  SumOutMax=[]  SumI1OutMin=[]  SumI1OutMax=[]  SumI2OutMin=[]  SumI2OutMax=[]  SumI3OutMin=[]  SumI3OutMax=[]  SumDOutMin=[]  SumDOutMax=[]  SaturationOutMin=[]  SaturationOutMax=[]  IntegratorContinuousStateAttributes=''  IntegratorStateMustResolveToSignalObject=off  IntegratorRTWStateStorageClass=Auto  FilterContinuousStateAttributes=''  FilterStateMustResolveToSignalObject=off  FilterRTWStateStorageClass=Auto  DifferentiatorICPrevScaledInput=0  DifferentiatorOutMin=[]  DifferentiatorOutMax=[]  FilterDiffOutCoefMin=[]  FilterDiffOutCoefMax=[]  SumDenOutMin=[]  SumDenOutMax=[]  SumNumOutMin=[]  SumNumOutMax=[]  ReciprocalOutMin=[]  ReciprocalOutMax=[]  DivideOutMin=[]  DivideOutMax=[]  TunerSelectOption=Transfer Function Based (PID Tuner App)
  PID Controller 0.15 : simulink/Continuous/PID Controller  Controller=PID  TimeDomain=Continuous-time  SampleTime=-1  IntegratorMethod=Forward Euler  FilterMethod=Forward Euler  Form=Parallel  UseFilter=on  ControllerParametersSource=internal  P=4  I=0  D=0  N=100  InitialConditionSource=internal  InitialConditionForIntegrator=0  InitialConditionForFilter=0  ExternalReset=none  LimitOutput=off  UpperSaturationLimit=inf  LowerSaturationLimit=-inf  LinearizeAsGain=on  AntiWindupMode=none  Kb=1  TrackingMode=off  Kt=1  PParamMin=[]  PParamMax=[]  IParamMin=[]  IParamMax=[]  DParamMin=[]  DParamMax=[]  NParamMin=[]  NParamMax=[]  KbParamMin=[]  KbParamMax=[]  KtParamMin=[]  KtParamMax=[]  POutMin=[]  POutMax=[]  IOutMin=[]  IOutMax=[]  DOutMin=[]  DOutMax=[]  NOutMin=[]  NOutMax=[]  KbOutMin=[]  KbOutMax=[]  KtOutMin=[]  KtOutMax=[]  IntegratorOutMin=[]  IntegratorOutMax=[]  FilterOutMin=[]  FilterOutMax=[]  SumOutMin=[]  SumOutMax=[]  SumI1OutMin=[]  SumI1OutMax=[]  SumI2OutMin=[]  SumI2OutMax=[]  SumI3OutMin=[]  SumI3OutMax=[]  SumDOutMin=[]  SumDOutMax=[]  SaturationOutMin=[]  SaturationOutMax=[]  IntegratorContinuousStateAttributes=''  IntegratorStateMustResolveToSignalObject=off  IntegratorRTWStateStorageClass=Auto  FilterContinuousStateAttributes=''  FilterStateMustResolveToSignalObject=off  FilterRTWStateStorageClass=Auto  DifferentiatorICPrevScaledInput=0  DifferentiatorOutMin=[]  DifferentiatorOutMax=[]  FilterDiffOutCoefMin=[]  FilterDiffOutCoefMax=[]  SumDenOutMin=[]  SumDenOutMax=[]  SumNumOutMin=[]  SumNumOutMax=[]  ReciprocalOutMin=[]  ReciprocalOutMax=[]  DivideOutMin=[]  DivideOutMax=[]  TunerSelectOption=Transfer Function Based (PID Tuner App)
  PID Controller 0.15 p : simulink/Continuous/PID Controller  Controller=PID  TimeDomain=Continuous-time  SampleTime=-1  IntegratorMethod=Forward Euler  FilterMethod=Forward Euler  Form=Parallel  UseFilter=on  ControllerParametersSource=internal  P=3  I=0  D=0  N=100  InitialConditionSource=internal  InitialConditionForIntegrator=0  InitialConditionForFilter=0  ExternalReset=none  LimitOutput=off  UpperSaturationLimit=inf  LowerSaturationLimit=-inf  LinearizeAsGain=on  AntiWindupMode=none  Kb=1  TrackingMode=off  Kt=1  PParamMin=[]  PParamMax=[]  IParamMin=[]  IParamMax=[]  DParamMin=[]  DParamMax=[]  NParamMin=[]  NParamMax=[]  KbParamMin=[]  KbParamMax=[]  KtParamMin=[]  KtParamMax=[]  POutMin=[]  POutMax=[]  IOutMin=[]  IOutMax=[]  DOutMin=[]  DOutMax=[]  NOutMin=[]  NOutMax=[]  KbOutMin=[]  KbOutMax=[]  KtOutMin=[]  KtOutMax=[]  IntegratorOutMin=[]  IntegratorOutMax=[]  FilterOutMin=[]  FilterOutMax=[]  SumOutMin=[]  SumOutMax=[]  SumI1OutMin=[]  SumI1OutMax=[]  SumI2OutMin=[]  SumI2OutMax=[]  SumI3OutMin=[]  SumI3OutMax=[]  SumDOutMin=[]  SumDOutMax=[]  SaturationOutMin=[]  SaturationOutMax=[]  IntegratorContinuousStateAttributes=''  IntegratorStateMustResolveToSignalObject=off  IntegratorRTWStateStorageClass=Auto  FilterContinuousStateAttributes=''  FilterStateMustResolveToSignalObject=off  FilterRTWStateStorageClass=Auto  DifferentiatorICPrevScaledInput=0  DifferentiatorOutMin=[]  DifferentiatorOutMax=[]  FilterDiffOutCoefMin=[]  FilterDiffOutCoefMax=[]  SumDenOutMin=[]  SumDenOutMax=[]  SumNumOutMin=[]  SumNumOutMax=[]  ReciprocalOutMin=[]  ReciprocalOutMax=[]  DivideOutMin=[]  DivideOutMax=[]  TunerSelectOption=Transfer Function Based (PID Tuner App)
  yaw rate : Outport
  wires:
  delta yaw/1 -> Cos/1  "delta yaw"
  Cos/1 -> Atan2/1
  PID Controller 0.075/1 -> yaw rate/1  "yaw rate"
  Atan2/1 -> PID Controller 0.075/1  "d yaw"
  Cos/2 -> Atan2/2

== system Bebop7_like6_but_spline_only_from_SP/Control/Orientation to 3D yaw rotation ==
  note: eul2rotm
  Drone yaw : Inport
  Constant1 : Constant  Value=0
  Rotation Angles to Direction Cosine Matrix : sharedtransform/Rotation Angles to Direction Cosine Matrix  rotationOrder=ZYX  aMode=aMode
      settings: SourceProductBaseCode=AE
  Vector Concatenate : Concatenate  NumInputs=3
  rot matrix : Outport
  wires:
  Constant1/1 -> Vector Concatenate/2, Vector Concatenate/3
  Vector Concatenate/1 -> Rotation Angles to Direction Cosine Matrix/1
  Drone yaw/1 -> Vector Concatenate/1  "yaw"
  Rotation Angles to Direction Cosine Matrix/1 -> rot matrix/1  "rot matrix"
